simulink model "rotpen_lqr_26"  (R2025a)
settings: Solver=ode45  StartTime=0.0  StopTime=run_time  RelTol=1e-3  EnableMultiTasking=on
values from neighbouring files (symbols this model uses):
  A = 0.2    [Multisine_test.m]    (also in compute_lqr.m = double(subs(subs(A_sym, x, x0), u, 0)); compute_mpc.m = double(subs(subs(A_sym, x, x0), u, 0)); link2_ode.m = [0 1; -beta -alpha]; my_pendulum_model.m = [0,  1,  0,  0)
  adingain = [adingain 1 1 1 1 1]    [hwinit.m]
  adinoffs = [adinoffs 0 0 0 0 0]    [hwinit.m]
  B = zeros(n, nu)    [Multisine_test.m]    (also in compute_lqr.m = double(subs(subs(B_sym, x, x0), u, 0)); compute_mpc.m = double(subs(subs(B_sym, x, x0), u, 0)); link2_ode.m = zeros(2, 0); my_pendulum_model.m = [0; b; 0; 0])
  C = [1 0 0 0 ... (first row only)    [Multisine_test.m]    (also in compute_lqr.m; compute_mpc.m; link2_ode.m = [1 0]; my_pendulum_model.m = eye(4))
  controller_sat = 1    [run_controller.m]    (also in run_freeswing.m = 0; run_lqr.m; run_mpc.m; run_ref_tracking.m)
  daoutgain = 1*[-6]    [hwinit.m]
  daoutoffs = [0.00]    [hwinit.m]
  h = 0.01    [Multisine_test.m]    (also in animate_pendulum.m = mean(diff(t)); collect_arm2_freeswing.m; collect_freeswing.m; first-script.m)
  K = lqr(A, B, Q, R)    [compute_lqr.m]    (also in link2_ode.m = zeros(2, 1); run_controller.m = K_full; run_ref_tracking.m = K_full(1:4))
  K_int = 0    [run_controller.m]    (also in run_ref_tracking.m = K_full(5))
  L = [31.5412926965  -1.46586450973  1.48832994181  104.88438352; 1.48832994181  0.281132012302  39.1187891696  266.247396057]    [lqr_gains.mat]
  offset = [pi; 0]    [run_controller.m]    (also in run_lqr.m; run_mpc.m; run_ref_tracking.m = [0; -pi])
  ref = [-pi; 0; 0; 0]    [run_controller.m]    (also in run_lqr.m = [pi; 0; 0; 0]; run_mpc.m = [pi; 0]; run_ref_tracking.m = ref_eq)
libraries: simulink_extras x1
settings Model: Creator=rbabuska  LastModifiedBy=thomas
settings SolverCC: AlgebraicLoopSolver=TrustRegion
settings DataIOCC: SaveFormat=Array  ReturnWorkspaceOutputs=off  SignalLoggingName=sigsOut
settings OptimizationCC: BooleanDataType=off  ExpressionDepthLimit=2147483647.0  InitFltsAndDblsToZero=on  LifeSpan=inf
settings DebuggingCC: SaveWithParameterizedLinksMsg=none  SignalResolutionControl=TryResolveAllWithWarning  MultiTaskDSMMsg=warning  MultiTaskCondExecSysMsg=none  UnconnectedInputMsg=warning  UnconnectedOutputMsg=warning  UnconnectedLineMsg=warning  AllowSymbolicDim=off  StateNameClashWarn=warning  SFUnexpectedBacktrackingDiag=warning  SFNoUnconditionalDefaultTransitionDiag=warning  SFExecutionAtInitializationDiag=none  ArithmeticOperatorsInVariantConditions=warning
settings HardwareCC: ProdBitPerPointer=32.0  ProdBitPerSizeT=32.0  ProdBitPerPtrDiffT=32.0  ProdLargestAtomicFloat=None  ProdIntDivRoundTo=Undefined  ProdEndianess=Unspecified  ProdWordSize=32.0  ProdHWDeviceType=32-bit Generic  TargetUnknown=on
settings ModelReferenceCC: EnableRefExpFcnMdlSchedulingChecks=on  PropagateSignalLabelsOutOfModel=off
settings SFSimCC: SimUseLocalCustomCode=off  CustomCodeUndefinedFunction=UseInterfaceOnly
settings RTWCC: RTWUseLocalCustomCode=off  GPUComputeCapability=3.5  DLArmComputeVersion=19.05
settings CodeAppCC: StateflowObjectComments=on
settings GRTTargetCC: TargetFcnLib=ansi_tfl_tmw.mat  TargetLangStandard=C89/C90 (ANSI)  CombineOutputUpdateFcns=off  GRTInterface=on
settings ConfigComp: CovMetricSettings=dw  CovSaveCumulativeToWorkspaceVar=on  CovSaveSingleToWorkspaceVar=on  CovExternalEMLEnable=off

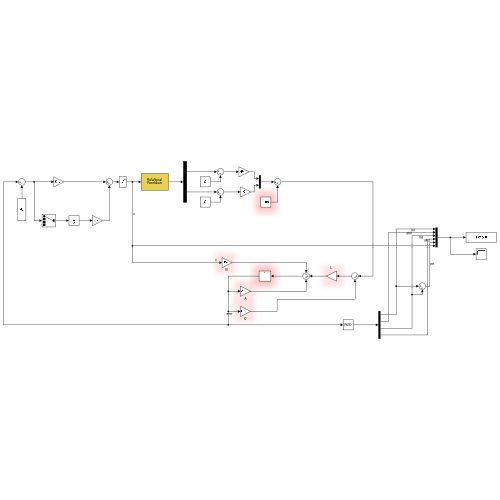
[thumbnail: Simulink's stored preview of the top-level diagram]
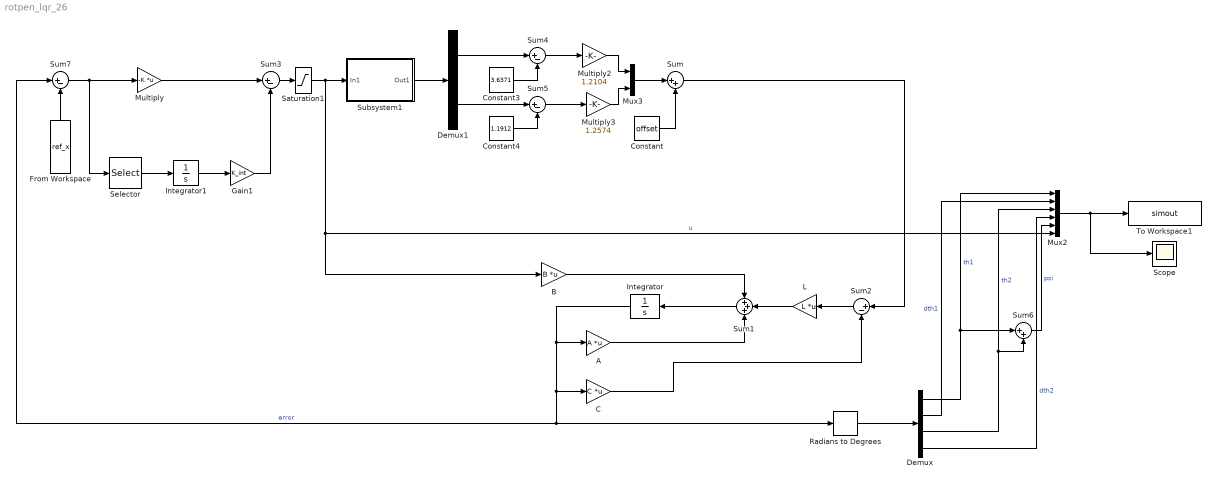
== system rotpen_lqr_26 ==
  A : Gain  Gain=A  Multiplication=Matrix(K*u)
  B : Gain  Gain=B  Multiplication=Matrix(K*u)
  C : Gain  Gain=C  Multiplication=Matrix(K*u)
  Constant : Constant  Value=offset
  Constant3 : Constant  Value=3.6371
  Constant4 : Constant  Value=1.1912
  Demux : Demux
  Demux1 : Demux  Outputs=2
  From Workspace : FromWorkspace  VariableName=ref_x
  Gain1 : Gain  Gain=K_int
  Integrator : Integrator  InitialCondition=0*ref
  Integrator1 : Integrator
  L : Gain  Gain=L  Multiplication=Matrix(K*u)
  Multiply : Gain  Gain=-K  Multiplication=Matrix(K*u)
  Multiply2 : Gain  Gain=1.2104
  Multiply3 : Gain  Gain=1.2574
  Mux2 : Mux  Inputs=6
  Mux3 : Mux  Inputs=2
  Radians to Degrees : simulink_extras/Transformations/Radians to Degrees
  Saturation1 : Saturate  UpperLimit=controller_sat  LowerLimit=-controller_sat
  Scope : Scope
      settings: ActiveDisplayYMinimum=-3.43648  ActiveDisplayYMaximum=2.90732
  Selector : Selector  InputPortWidth=4  IndexOptions=Index vector (dialog)  Indices=[1]  OutputSizes=1
  Subsystem1 : Subsystem
      mask Display: disp('Rotational\nPendulum')
  Sum : Sum  Inputs=|++
  Sum1 : Sum  Inputs=+++
  Sum{2..5,7} (5 alike) : Sum  Inputs=|+-
  Sum6 : Sum  Inputs=|++
  To Workspace1 : ToWorkspace  VariableName=simout  SaveFormat=Timeseries  SampleTime=-1
  wires:
  Constant3/1 -> Sum4/2
  Mux2/1 -> To Workspace1/1, Scope/1
  Sum5/1 -> Multiply3/1
  Sum4/1 -> Multiply2/1
  Demux1/1 -> Sum4/1
  Constant4/1 -> Sum5/2
  Demux1/2 -> Sum5/1
  Saturation1/1 -> Subsystem1/1(In1), Mux2/6, B/1  "u"
  Subsystem1/1(Out1) -> Demux1/1
  Integrator/1 -> A/1, Sum7/1, Radians to Degrees/1, C/1  "error"
  B/1 -> Sum1/1
  Sum1/1 -> Integrator/1
  A/1 -> Sum1/3
  L/1 -> Sum1/2
  Demux/1 -> Sum6/1, Mux2/1  "th1"
  Demux/2 -> Mux2/2  "dth1"
  Demux/3 -> Sum6/2, Mux2/3  "th2"
  Demux/4 -> Mux2/4  "dth2"
  Sum2/1 -> L/1
  C/1 -> Sum2/2
  Radians to Degrees/1 -> Demux/1
  Multiply2/1 -> Mux3/1
  Multiply3/1 -> Mux3/2
  Mux3/1 -> Sum/1
  Constant/1 -> Sum/2
  Sum/1 -> Sum2/1
  Multiply/1 -> Sum3/1
  Sum6/1 -> Mux2/5  "psi"
  Sum3/1 -> Saturation1/1
  Selector/1 -> Integrator1/1
  Integrator1/1 -> Gain1/1
  Gain1/1 -> Sum3/2
  From Workspace/1 -> Sum7/2
  Sum7/1 -> Selector/1, Multiply/1

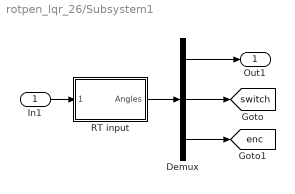
== system rotpen_lqr_26/Subsystem1 ==
  In1 : Inport
  Demux : Demux  Outputs=[2 4 1]
  RT input : Subsystem  mask{Ts=h, channels=[6 7]}
      mask prompts: Ts "Sample time [s]:"; channels "Channels to read (e.g., [6 7])"
      mask init:
      | hwinit;
      | 
      | % initialize FPGA
      | fugihandle = fugiboard('Open', 'Pendulum1');
      | fugihandle.WatchdogTimeout = 0.5;
      | fugiboard('SetParams', fugihandle);
      | fugiboard('Write', fugihandle, 0, 0, 0, 0);  % dummy write to sync interface board
      | fugiboard('Write', fugihandle, 5, 1, 0, 0);  % reset position, activate relay
      | data = fugiboard('Read', fugihandle);        % get version info from FPGA
      | % model = bitshift(data(1), -5); 
      | % version = bitand(data(1), 31);
      | % disp(sprintf('FPGA setup %d, version %d', model, version)); % for the B&P it should say 1 1, or else there is a problem
      | fugiboard('Write', fugihandle, 0, 1, 0, 0);  % end reset
      | pause(0.1);                         % give relay some time to respond
      mask Display: disp('Rotational\nPendulum')
  Out1 : Outport
  tag scope: enc=global, switch=global
  wires:
  RT input/1(Angles) -> Demux/1
  Demux/1 -> Out1/1
  In1/1 -> RT input/1(Motors)
  Demux/2 -> [switch]
  Demux/3 -> [enc]

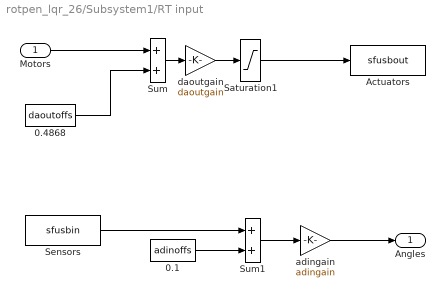
== system rotpen_lqr_26/Subsystem1/RT input ==
  Motors : Inport
  0.1 : Constant  Value=adinoffs
  0.4868 : Constant  Value=daoutoffs
  Actuators : S-Function  FunctionName=sfusbout  Parameters=Ts, fugihandle  SFunctionDeploymentMode=off  EnableBusSupport=off
  Saturation1 : Saturate  UpperLimit=10  LowerLimit=-10
  Sensors : S-Function  FunctionName=sfusbin  Parameters=Ts, fugihandle, channels  SFunctionDeploymentMode=off  EnableBusSupport=off
  Sum : Sum  InputSameDT=on  SaturateOnIntegerOverflow=on  OutDataTypeStr=Inherit: Same as first input
  Sum1 : Sum  InputSameDT=on  SaturateOnIntegerOverflow=on  OutDataTypeStr=Inherit: Same as first input
  adingain : Gain  Gain=adingain  SaturateOnIntegerOverflow=on  OutDataTypeStr=Inherit: Same as input  ParamDataTypeStr=Inherit: Same as input
  daoutgain : Gain  Gain=daoutgain  SaturateOnIntegerOverflow=on  OutDataTypeStr=Inherit: Same as input  ParamDataTypeStr=Inherit: Same as input
  Angles : Outport
  wires:
  Sum/1 -> daoutgain/1
  0.4868/1 -> Sum/2
  Motors/1 -> Sum/1
  Sum1/1 -> adingain/1
  0.1/1 -> Sum1/2
  adingain/1 -> Angles/1
  Saturation1/1 -> Actuators/1
  daoutgain/1 -> Saturation1/1
  Sensors/1 -> Sum1/1
